simulink model "Elicottero2DOF_Sim"  (R2025b)
settings: Solver=VariableStepAuto  StartTime=0.0  StopTime=20  FixedStep=0.0005  RelTol=1e-3
values from neighbouring files (symbols this model uses):
  F1 = 0.5    [Elicottero2DOF_INIT.m]
  F2 = 0    [Elicottero2DOF_INIT.m]
  M_0 = 46.5    [Elicottero2DOF_INIT.m]
  MAHALANOBIS = true    [Elicottero2DOF_INIT.m]
  Outlier_flag = 1    [Elicottero2DOF_INIT.m]
  P0 = diag([P_0_alpha P_0_alpha_dot P_0_beta P_0_beta_dot])    [Elicottero2DOF_INIT.m]
  q_0 = [alpha_0 beta_0]'    [Elicottero2DOF_INIT.m]
  q_dot_0 = [alpha_dot_0 beta_dot_0]'    [Elicottero2DOF_INIT.m]
  seme_rumore = 12345    [Elicottero2DOF_INIT.m]
  sigma_acc = 0.0137    [Elicottero2DOF_INIT.m]
  sigma_magn = 0.14    [Elicottero2DOF_INIT.m]
  st_acc = 0.00435    [Elicottero2DOF_INIT.m]
  st_magn = 0.005    [Elicottero2DOF_INIT.m]
  x_0 = [0 0 0 0]'    [Elicottero2DOF_INIT.m]
undefined symbols (not defined in the file or in its folder): params
libraries: simulink x2
settings Model: Creator=giggi  LastModifiedBy=giggi

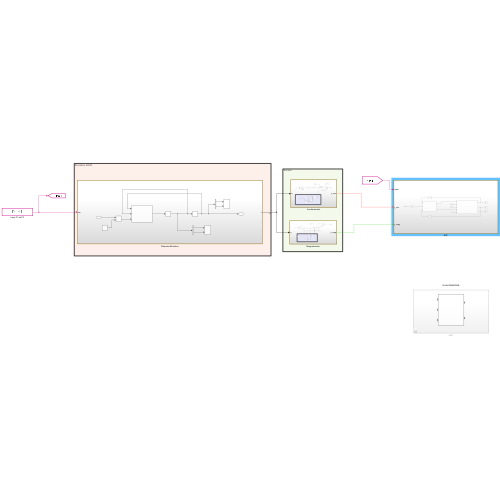
[thumbnail: Simulink's stored preview of the top-level diagram]
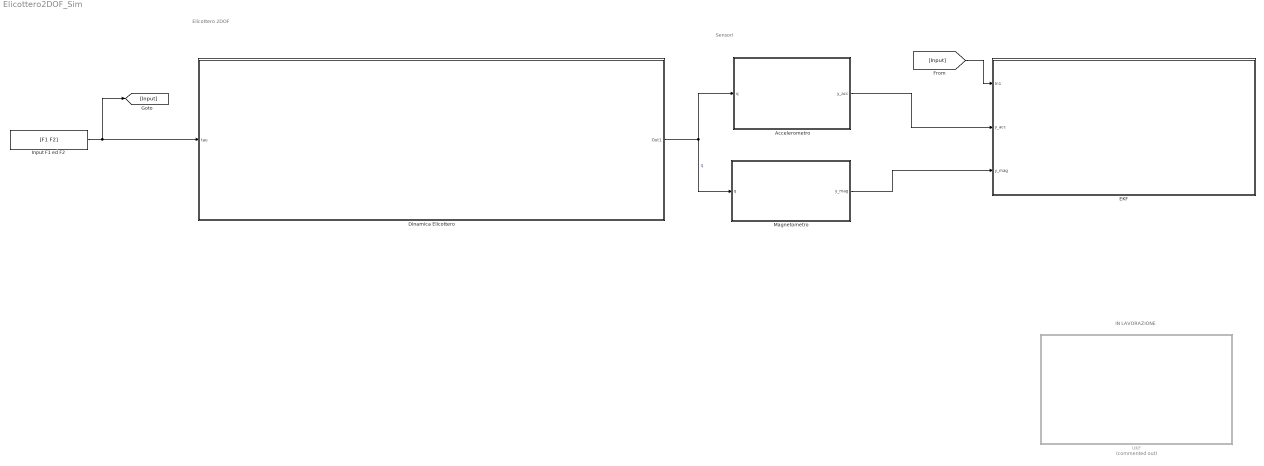
== system Elicottero2DOF_Sim ==
  note: IN LAVORAZIONE
  note: Elicottero 2DOF
  note: Sensori
  Accelerometro : Subsystem
  Dinamica Elicottero : Subsystem
  EKF : Subsystem
  Input F1 ed F2 : Constant  Value=[F1 F2]
  Magnetometro : Subsystem
  UKF : Subsystem  Commented=on
  wires:
  Input F1 ed F2/1 -> Dinamica Elicottero/1(tau), [Input]
  Dinamica Elicottero/1(Out1) -> Magnetometro/1(q), Accelerometro/1(q)  "q"
  [Input] -> EKF/1(In1)
  Accelerometro/1(y_acc) -> EKF/2(y_acc)
  Magnetometro/1(y_mag) -> EKF/3(y_mag)

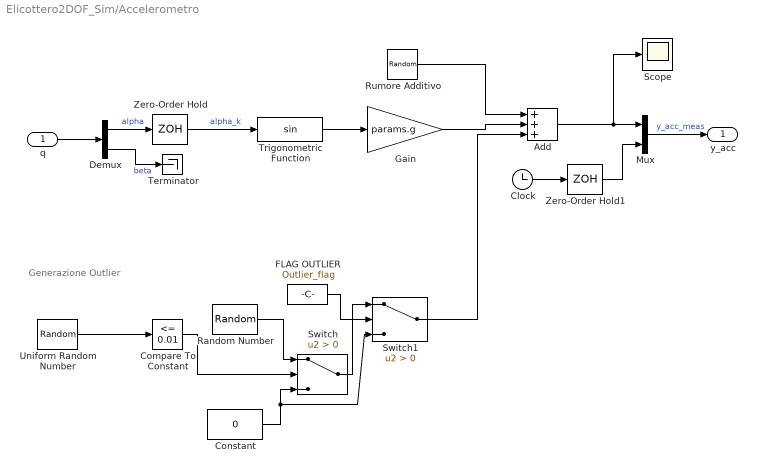
== system Elicottero2DOF_Sim/Accelerometro ==
  note: Generazione Outlier
  q : Inport
  Add : Sum  Inputs=+++
  Clock : Clock
  Compare To Constant : simulink/Logic and Bit Operations/Compare To Constant  relop=<=  const=0.01  OutDataTypeStr=boolean
  Constant : Constant  Value=0  SampleTime=st_acc
  Demux : Demux  Outputs=2
  FLAG OUTLIER : Constant  Value=Outlier_flag  SampleTime=st_acc
  Gain : Gain  Gain=params.g
  Mux : Mux  Inputs=2
  Random Number : RandomNumber  Variance=100  Seed=seme_rumore + 18  SampleTime=st_acc
  Rumore Additivo : RandomNumber  Variance=sigma_acc^2  Seed=seme_rumore  SampleTime=st_acc
  Scope : Scope
      settings: ActiveDisplayYMinimum=-30.088997858542836  ActiveDisplayYMaximum=33.1256414934188
  Switch : Switch  Criteria=u2 > Threshold  SaturateOnIntegerOverflow=off  InputSameDT=off
  Switch1 : Switch  Criteria=u2 > Threshold  SaturateOnIntegerOverflow=off  InputSameDT=off
  Terminator : Terminator
  Trigonometric Function : Trigonometry
  Uniform Random Number : UniformRandomNumber  Minimum=0  Seed=seme_rumore + 953  SampleTime=st_acc
  Zero-Order Hold : ZeroOrderHold  SampleTime=st_acc
  Zero-Order Hold1 : ZeroOrderHold  SampleTime=st_acc
  y_acc : Outport
  wires:
  q/1 -> Demux/1
  Demux/1 -> Zero-Order Hold/1  "alpha"
  Demux/2 -> Terminator/1  "beta"
  Trigonometric Function/1 -> Gain/1
  Gain/1 -> Add/2
  Rumore Additivo/1 -> Add/1
  Add/1 -> Mux/1, Scope/1
  Zero-Order Hold/1 -> Trigonometric Function/1  "alpha_k"
  Mux/1 -> y_acc/1  "y_acc_meas"
  Clock/1 -> Zero-Order Hold1/1
  Zero-Order Hold1/1 -> Mux/2
  FLAG OUTLIER/1 -> Switch1/2
  Constant/1 -> Switch1/3, Switch/3
  Compare To Constant/1 -> Switch/2
  Random Number/1 -> Switch/1
  Switch/1 -> Switch1/1
  Switch1/1 -> Add/3
  Uniform Random Number/1 -> Compare To Constant/1

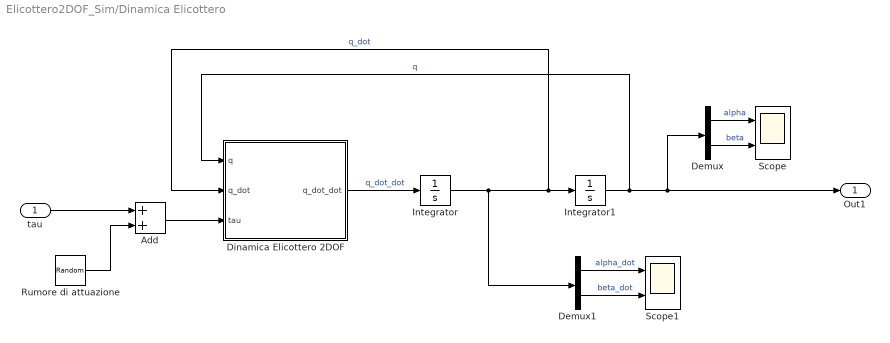
== system Elicottero2DOF_Sim/Dinamica Elicottero ==
  tau : Inport
  Add : Sum
  Demux : Demux  Outputs=2
  Demux1 : Demux  Outputs=2
  Dinamica Elicottero 2DOF : MATLAB Function  TreatAsAtomicUnit=on
  Integrator : Integrator  InitialCondition=q_dot_0
  Integrator1 : Integrator  InitialCondition=q_0
  Rumore di attuazione : RandomNumber  Mean=[0 0]  Variance=[params.sigma_F params.sigma_F].^2  Seed=seme_rumore + 15  SampleTime=params.st
  Scope : Scope  NumInputPorts=2
      settings: ActiveDisplayYMinimum=-0.16061252494625422  ActiveDisplayYMaximum=1.8001420960767636
  Scope1 : Scope  NumInputPorts=2
      settings: ActiveDisplayYMinimum=-0.1165873755543972  ActiveDisplayYMaximum=0.333104748254671  DataLoggingVariableName=ScopeData4
  Out1 : Outport
  wires:
  Demux/1 -> Scope/1  "alpha"
  Integrator1/1 -> Out1/1, Demux/1, Dinamica Elicottero 2DOF/1(q)  "q"
  Dinamica Elicottero 2DOF/1(q_dot_dot) -> Integrator/1  "q_dot_dot"
  Demux/2 -> Scope/2  "beta"
  Demux1/1 -> Scope1/1  "alpha_dot"
  Demux1/2 -> Scope1/2  "beta_dot"
  Integrator/1 -> Demux1/1, Dinamica Elicottero 2DOF/2(q_dot), Integrator1/1  "q_dot"
  tau/1 -> Add/1
  Add/1 -> Dinamica Elicottero 2DOF/3(tau)
  Rumore di attuazione/1 -> Add/2

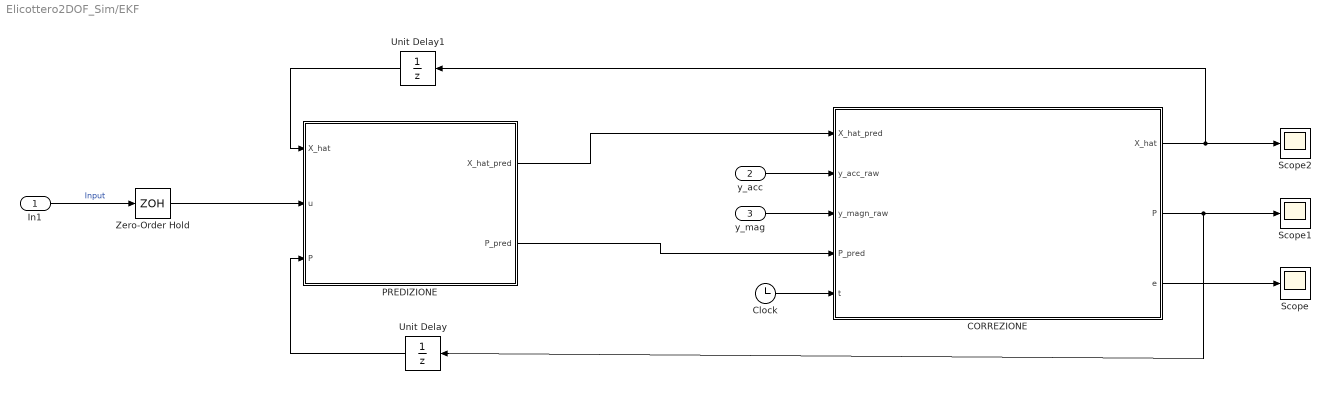
== system Elicottero2DOF_Sim/EKF ==
  In1 : Inport
  y_acc : Inport  Port=2
  y_mag : Inport  Port=3
  CORREZIONE : MATLAB Function  TreatAsAtomicUnit=on
  Clock : Clock
  PREDIZIONE : MATLAB Function  TreatAsAtomicUnit=on
  Scope : Scope
      settings: ActiveDisplayYMinimum=-0.065274363469370072  ActiveDisplayYMaximum=0.060684676727098576  DataLoggingVariableName=ScopeData6
  Scope1 : Scope
      settings: ActiveDisplayYMinimum=-1  ActiveDisplayYMaximum=1  DataLoggingVariableName=ScopeData5
  Scope2 : Scope
      settings: ActiveDisplayYMinimum=-5.8937824118242137  ActiveDisplayYMaximum=6.6213179612778612  DataLoggingVariableName=ScopeData7
  Unit Delay : UnitDelay  InitialCondition=P0  SampleTime=params.st  HasFrameUpgradeWarning=on
  Unit Delay1 : UnitDelay  InitialCondition=x_0  SampleTime=params.st  HasFrameUpgradeWarning=on
  Zero-Order Hold : ZeroOrderHold  SampleTime=params.st
  wires:
  PREDIZIONE/2(P_pred) -> CORREZIONE/4(P_pred)
  Zero-Order Hold/1 -> PREDIZIONE/2(u)
  In1/1 -> Zero-Order Hold/1  "Input"
  Unit Delay/1 -> PREDIZIONE/3(P)
  Unit Delay1/1 -> PREDIZIONE/1(X_hat)
  y_acc/1 -> CORREZIONE/2(y_acc_raw)
  y_mag/1 -> CORREZIONE/3(y_magn_raw)
  CORREZIONE/1(X_hat) -> Unit Delay1/1, Scope2/1
  PREDIZIONE/1(X_hat_pred) -> CORREZIONE/1(X_hat_pred)
  CORREZIONE/2(P) -> Unit Delay/1, Scope1/1
  Clock/1 -> CORREZIONE/5(t)
  CORREZIONE/3(e) -> Scope/1

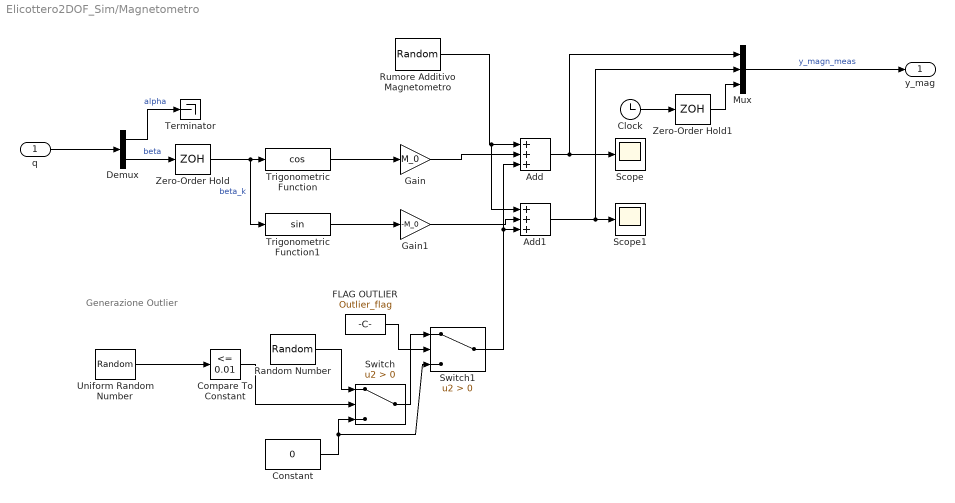
== system Elicottero2DOF_Sim/Magnetometro ==
  note: Generazione Outlier
  q : Inport
  Add : Sum  Inputs=+++
  Add1 : Sum  Inputs=+++
  Clock : Clock
  Compare To Constant : simulink/Logic and Bit Operations/Compare To Constant  relop=<=  const=0.01  OutDataTypeStr=boolean
  Constant : Constant  Value=0  SampleTime=st_magn
  Demux : Demux  Outputs=2
  FLAG OUTLIER : Constant  Value=Outlier_flag  SampleTime=st_magn
  Gain : Gain  Gain=M_0
  Gain1 : Gain  Gain=-M_0
  Mux : Mux  Inputs=3
  Random Number : RandomNumber  Variance=100  Seed=seme_rumore + 43  SampleTime=st_magn
  Rumore Additivo Magnetometro : RandomNumber  Variance=sigma_magn^2  Seed=seme_rumore + 1  SampleTime=st_magn
  Scope : Scope
      settings: ActiveDisplayYMinimum=-9.5570732834718957  ActiveDisplayYMaximum=53.128042723448729  DataLoggingVariableName=ScopeData2
  Scope1 : Scope
      settings: ActiveDisplayYMinimum=-1  ActiveDisplayYMaximum=1  DataLoggingVariableName=ScopeData3
  Switch : Switch  Criteria=u2 > Threshold  SaturateOnIntegerOverflow=off  InputSameDT=off
  Switch1 : Switch  Criteria=u2 > Threshold  SaturateOnIntegerOverflow=off  InputSameDT=off
  Terminator : Terminator
  Trigonometric Function : Trigonometry  Operator=cos
  Trigonometric Function1 : Trigonometry
  Uniform Random Number : UniformRandomNumber  Minimum=0  Seed=seme_rumore + 921  SampleTime=st_magn
  Zero-Order Hold : ZeroOrderHold  SampleTime=st_magn
  Zero-Order Hold1 : ZeroOrderHold  SampleTime=st_magn
  y_mag : Outport
  wires:
  q/1 -> Demux/1
  Demux/2 -> Zero-Order Hold/1  "beta"
  Demux/1 -> Terminator/1  "alpha"
  Trigonometric Function/1 -> Gain/1
  Trigonometric Function1/1 -> Gain1/1
  Gain/1 -> Add/2
  Rumore Additivo Magnetometro/1 -> Add1/1, Add/1
  Gain1/1 -> Add1/2
  Add/1 -> Mux/1, Scope/1
  Add1/1 -> Mux/2, Scope1/1
  Zero-Order Hold/1 -> Trigonometric Function1/1, Trigonometric Function/1  "beta_k"
  Mux/1 -> y_mag/1  "y_magn_meas"
  Clock/1 -> Zero-Order Hold1/1
  Zero-Order Hold1/1 -> Mux/3
  Uniform Random Number/1 -> Compare To Constant/1
  Random Number/1 -> Switch/1
  Compare To Constant/1 -> Switch/2
  Constant/1 -> Switch1/3, Switch/3
  FLAG OUTLIER/1 -> Switch1/2
  Switch/1 -> Switch1/1
  Switch1/1 -> Add/3, Add1/3

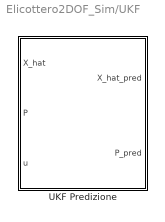
== system Elicottero2DOF_Sim/UKF ==
  UKF Predizione : MATLAB Function  TreatAsAtomicUnit=on

== matlab function Elicottero2DOF_Sim/EKF/PREDIZIONE ==
  data: X_hat input; u input; P input; X_hat_pred output; P_pred output; params parameter
function [X_hat_pred, P_pred] = Predizione(X_hat, u, P, params)
    % PREDIZIONE EKF - Modello con Rumore di Attuazione sui Motori
    
    %% 1. Lettura dello Stato e Ingressi
    alpha     = X_hat(1);
    alpha_dot = X_hat(2);
    beta      = X_hat(3);
    beta_dot  = X_hat(4);
    
    F1 = u(1);
    F2 = u(2);
    
    %% 2. Estrazione Parametri Fisici
    m  = params.m;       l  = params.l;       g  = params.g;
    Ja = params.J_alpha; Jy = params.J_y;     Jz = params.J_z;
    Ib = params.I_b;     ca = params.c_alpha; cb = params.c_beta;
    ep = params.epsilon_p;   ey = params.epsilon_y;   
    dt = params.st;
    
    %% 3. Matrice di Covarianza del Rumore di Processo (Q)
    % Q è 2x2. Contiene la varianza del rumore dei motori EMAX MT2204
    % param.sigma_F = 0.05 [Newton]
    Q = [params.sigma_F^2, 0;
         0,               params.sigma_F^2];

    %% 4. MODELLO DINAMICO NON LINEARE
    J_beta = Jy * sin(alpha)^2 + (Jz + m*l^2) * cos(alpha)^2 + Ib;
    
    alpha_ddot = (-ca * alpha_dot - m * g * l * sin(alpha) + ...
                   l * F1 * cos(beta) + ep * l * F2 * sin(beta)) / Ja;
                   
    beta_ddot  = (-cb * beta_dot + l * F2 * cos(alpha) + ...
                   ey * l * F1 * sin(alpha)) / J_beta;

    %% 5. PREDIZIONE DELLO STATO (Eulero)
    X_hat_pred = [alpha     + dt * alpha_dot;
                  alpha_dot + dt * alpha_ddot;
                  beta      + dt * beta_dot;
                  beta_dot  + dt * beta_ddot];

    %% 6. CALCOLO JACOBIANA DI PROCESSO (A) -> F = I + A*dt
    % Derivate per la riga 2 (alpha_ddot)
    A21 = (-m * g * l * cos(alpha)) / Ja;
    A22 = -ca / Ja;
    A23 = (-l * F1 * sin(beta) + ep * l * F2 * cos(beta)) / Ja;
    A24 = 0;
    
    % Derivate per la riga 4 (beta_ddot)
    N = -cb * beta_dot + l * F2 * cos(alpha) + ey * l * F1 * sin(alpha);
    D_den = J_beta;
    dN_dalpha = -l * F2 * sin(alpha) + ey * l * F1 * cos(alpha);
    dD_dalpha = 2 * Jy * sin(alpha) * cos(alpha) - 2 * (Jz + m*l^2) * cos(alpha) * sin(alpha);
    
    A41 = (D_den * dN_dalpha - N * dD_dalpha) / (D_den^2);
    A42 = 0;
    A43 = 0;
    A44 = -cb / D_den;
    
    % Assemblaggio e discretizzazione
    A = [  0,   1,   0,   0;
         A21, A22, A23, A24;
           0,   0,   0,   1;
         A41, A42, A43, A44];
         
    F = eye(4) + A * dt;
    
    %% 7. CALCOLO JACOBIANA DEI DISTURBI (D)
    % Rappresenta l'impatto di 1 Newton di errore del motore sulle accelerazioni.
    % La matrice è 4x2 perché mappa 2 rumori su 4 stati.
    
    d_alpha_ddot_w1 = (l * cos(beta)) / Ja;
    d_alpha_ddot_w2 = (ep * l * sin(beta)) / Ja;
    
    d_beta_ddot_w1  = (ey * l * sin(alpha)) / J_beta;
    d_beta_ddot_w2  = (l * cos(alpha)) / J_beta;
    
    D = [0,                         0;
         d_alpha_ddot_w1 * dt,      d_alpha_ddot_w2 * dt;
         0,                         0;
         d_beta_ddot_w1 * dt,       d_beta_ddot_w2 * dt];
         
    %% 8. PREDIZIONE DELLA COVARIANZA
    % Diffusione dell'incertezza dei motori negli stati tramite la matrice D
    P_pred = F * P * F' + D * Q * D';
    
end

== matlab function Elicottero2DOF_Sim/Dinamica Elicottero/Dinamica Elicottero 2DOF ==
  data: q input; q_dot input; tau input; q_dot_dot output; params parameter
function q_dot_dot = fcn(q, q_dot, tau, params)

alpha = q(1);
alpha_dot = q_dot(1);
beta = q(2);
beta_dot = q_dot(2);

% Costruzione Momento di Inerzia di Yaw (Variabile con angolo di pitch)
J_beta = params.J_y * sin(alpha)^2 + (params.J_z + params.m * params.l^2) * cos(alpha)^2 + params.I_b;

% Matrice di Inerzia
M = [params.J_alpha 0; 0 J_beta];

% Vettore dei termini non lineari (raccoglie attriti viscosi e forza di gravità)
n = [params.c_alpha * alpha_dot + params.m * params.g * params.l * sin(alpha); params.c_beta * beta_dot];

% Vettore delle Forze / Coppie generalizzate
B = [params.l * cos(beta), params.epsilon_p * params.l * sin(beta); params.epsilon_y * params.l * sin(alpha), params.l * cos(alpha)];

% Dinamica Inversa
q_dot_dot = M \ (B * tau - n);

== matlab function Elicottero2DOF_Sim/EKF/CORREZIONE ==
  data: X_hat_pred input; y_acc_raw input; y_magn_raw input; X_hat output; P_pred input; P output; params parameter; t input; MAHALANOBIS parameter; M_0 parameter; e output
function [X_hat, P, e] = Correzione(X_hat_pred, y_acc_raw, y_magn_raw, P_pred, params, t, MAHALANOBIS, M_0)
    % FUNZIONE DI CORREZIONE EKF 
    % Modello di osservazione: 
    % y_acc = gsin(alpha_k) + v_alpha_k
    % y_magn = [M_0*cos*(beta_k),-M_0*sin(beta_k)] + [v_beta_k, v_beta_k]

    g = params.g;
    dt = params.st;

    % Inizializzazione di sicurezza: se il filtro fa "return", 
    % restituisce la predizione intatta senza andare in crash.
    X_hat = X_hat_pred;
    P = P_pred;
    
    % Input (x_k|k-1)
    alpha = X_hat_pred(1); 
    beta = X_hat_pred(3);

    % Treshold per distanza di Mahalanobis
    mahalanobis_treshold = 3;

    % Uscite Sensori
    t_acc = y_acc_raw(2);
    t_magn = y_magn_raw(3);
    y_acc = y_acc_raw(1);
    y_magn = y_magn_raw(1:2);

      
    % Covarianze errore di misura
    R = diag([params.R_acc, params.R_magn, params.R_magn]);
    
    % Matrice M = dh_k/dv_k  valutata in x_k|k-1
    M = eye(3);

    % Matrice H = dh_k/x_k valutata in x_k|k-1
    H = [g*cos(alpha), 0, 0, 0; ...
        0, 0, -M_0*sin(beta), 0; ...
        0, 0, -M_0*cos(beta), 0];

    % Innovazione
    e = [y_acc; y_magn] - [g*sin(alpha); M_0*cos(beta);-M_0*sin(beta)];

    % Calcolo delle singole distanze di mahalanobis
    H_acc = H(1, :);
    e_acc = e(1);
    M_acc = M(1, 1);
    R_acc = R(1, 1);
    S_acc = H_acc * P_pred * H_acc' + M_acc * R_acc * M_acc';
    mahalanobis_acc = sqrt(e_acc' / S_acc * e_acc);

    H_magn = H(2:3, :);
    e_magn = e(2:3);
    M_magn = M(2:3, 2:3);
    R_magn = R(2:3, 2:3);
    S_magn = H_magn * P_pred * H_magn' + M_magn * R_magn * M_magn';
    mahalanobis_magn = sqrt(e_magn' / S_magn * e_magn);

    % Verifica della disponibilità delle misure
    if MAHALANOBIS
        flag_acc = (mahalanobis_acc <= mahalanobis_treshold) && (t_acc <= t) && (t - dt < t_acc);
        flag_magn = (mahalanobis_magn <= mahalanobis_treshold) && (t_magn <= t) && (t - dt < t_magn);
    else
        flag_acc =  (t_acc <= t) && (t - dt < t_acc);
        flag_magn = (t_magn <= t) && (t - dt < t_magn);
    end
   

    % Costruzione delle matrici in base alle misure valide
    % Entrambe le misure valide
    if flag_acc && flag_magn
        H_curr = H;
        e_curr = e;
        M_curr = M;
        R_curr = R;

    elseif flag_acc     % Solo misura accelerometro disponibile
        H_curr = H_acc;
        e_curr = e_acc;
        M_curr = M_acc;
        R_curr = R_acc;

    elseif flag_magn    % Solo misura magnetometro disponibile
        H_curr = H_magn;
        e_curr = e_magn;
        M_curr = M_magn;
        R_curr = R_magn;

    else                % Nessuna misura disponibile
        return;
    end

    % Covarianza dell'innovazione
    S = H_curr * P_pred * H_curr' + M_curr * R_curr * M_curr';

    % Guadagno di Correzione
    L = P_pred * H_curr' / S;
    
    % Aggiornamento stato e covarianza
    X_hat = X_hat_pred + L * e_curr;
    % Forma di Joseph
    P = (eye(4) - L * H_curr) * P_pred * (eye(4) - L * H_curr)' + L * R_curr * L';

end

== matlab function Elicottero2DOF_Sim/UKF/UKF Predizione ==
  data: X_hat input; X_hat_pred output; P input; P_pred output; params parameter; u input
function [X_hat_pred, P_pred] = UKF_Predizione(X_hat, P, params, u)

lambda = params.lambda;
n = params.n;

F1 = u(1);
F2 = u(2);

% Inizializzazione vettore sigma_points
sigma_points = zeros(n, 2*n + 1);

% Fattorizzazione di Cholesky covarianza
GAMMA = chol(P, 'lower');

% Estrazione Sigma-points(da -n ad n)
for i =-n:n
    idx = i + n + 1;
    if i == 0      
        sigma_points(:, idx) = X_hat;       % Sigma-point centrale
    elseif i < 0
        sigma_points(:, idx) = X_hat -sqrt(n + lambda) * GAMMA(:, i);
    elseif i > 0
        sigma_points(:, idx) = X_hat + sqrt(n + lambda) * GAMMA(:, abs(i));
    end
end


%--------------------------------------------------------------------------
% PROPAGAZIONE SIGMA-POINTS
%--------------------------------------------------------------------------

sigma_points_pred = zeros(n, 2*n + 1);






y = u;
